simulink model "MAS_new"  (R2023a)
settings: Solver=VariableStepAuto  StartTime=0.0  StopTime=1  RelTol=1e-3
values from neighbouring files (symbols this model uses):
  abc_alpha_beta = sqrt(2/3) * [1, -1/2, -1/2 ... (first row only)    [main.m]
  Flux_1 = 1/(Msr^2 - Ls * Lr )  * [Rs*Lr, 0, -Rs*Msr, 0 ... (first row only)    [main.m]
  Flux_2 = 1/(Msr^2 - Ls * Lr )  * [0, 0, 0, 0 ... (first row only)    [main.m]
  frot = 0.01    [main.m]
  Inv_abc_alpha_beta = inv(abc_alpha_beta)    [main.m]
  Inv_Phi_Courant = inv(Phi_Courant)    [main.m]
  J = 0.025    [main.m]
  Lr = 0.194    [main.m]
  Ls = 0.182    [main.m]
  Msr = 0.182    [main.m]
  p = 2    [main.m]
  T_charge = 0    [main.m]
  Vn = 380    [main.m]
settings Model: Creator=philippecasteres  LastModifiedBy=philippecasteres

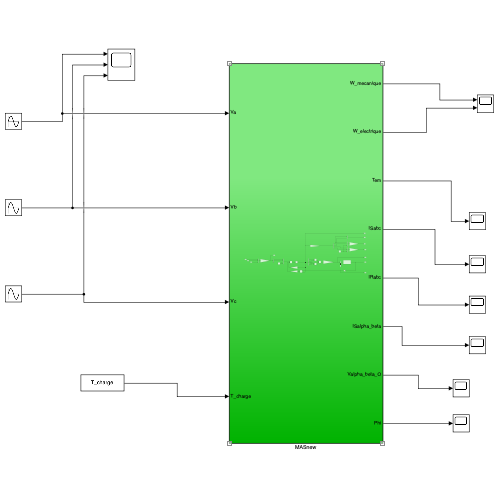
[thumbnail: Simulink's stored preview of the top-level diagram]
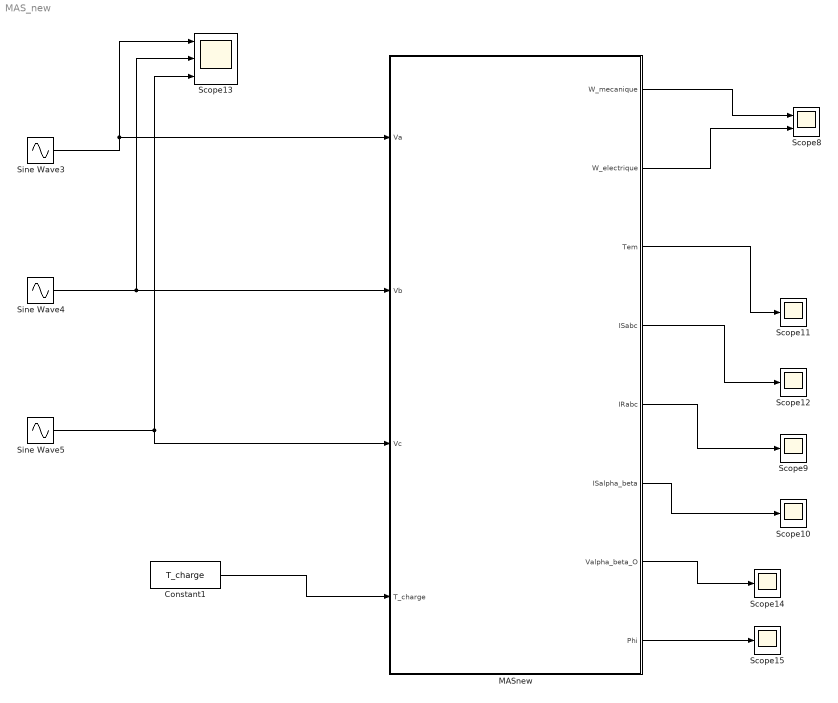
== system MAS_new ==
  Constant1 : Constant  Value=T_charge
  MASnew : Subsystem
  Scope{9..12,14..15} (6 alike) : Scope
  Scope13 : Scope  NumInputPorts=3
  Scope8 : Scope  NumInputPorts=2
  Sine Wave3 : Sin  Amplitude=Vn  Frequency=50*2*pi  SampleTime=0
  Sine Wave4 : Sin  Amplitude=Vn  Frequency=50*2*pi  Phase=-2*pi/3  SampleTime=0
  Sine Wave5 : Sin  Amplitude=Vn  Frequency=50*2*pi  Phase=-4*pi/3  SampleTime=0
  wires:
  MASnew/1(W_mecanique) -> Scope8/1
  MASnew/7(Valpha_beta_O) -> Scope14/1
  Sine Wave4/1 -> Scope13/2, MASnew/2(Vb)
  Sine Wave5/1 -> Scope13/3, MASnew/3(Vc)
  MASnew/6(ISalpha_beta) -> Scope10/1
  MASnew/8(Phi) -> Scope15/1
  MASnew/5(IRabc) -> Scope9/1
  MASnew/3(Tem) -> Scope11/1
  MASnew/4(ISabc) -> Scope12/1
  Sine Wave3/1 -> MASnew/1(Va), Scope13/1
  MASnew/2(W_electrique) -> Scope8/2
  Constant1/1 -> MASnew/4(T_charge)

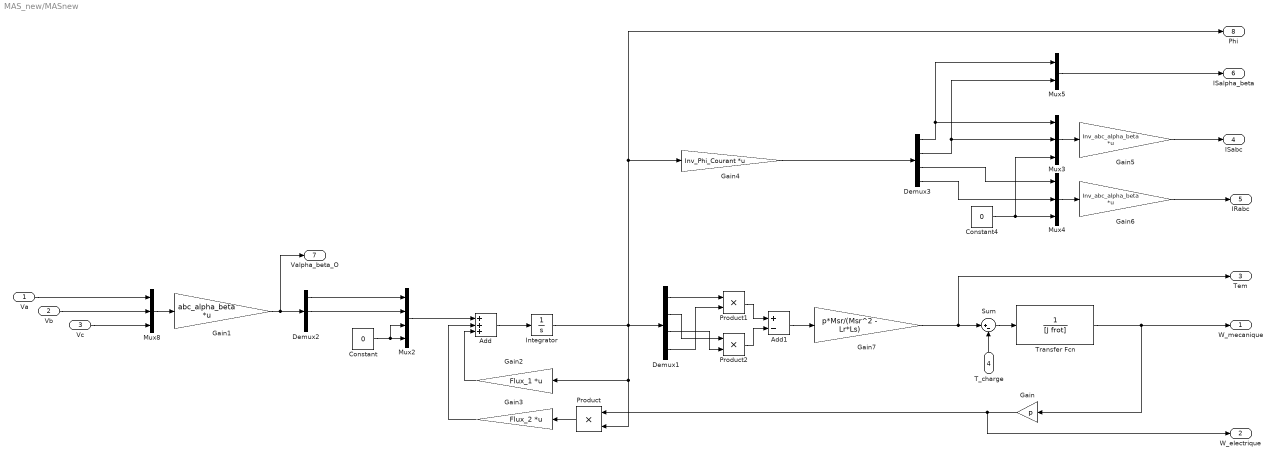
== system MAS_new/MASnew ==
  Va : Inport
  Vb : Inport  Port=2
  Vc : Inport  Port=3
  T_charge : Inport  Port=4
  Add : Sum  Inputs=+++
  Add1 : Sum  Inputs=+-
  Constant : Constant  Value=0
  Constant4 : Constant  Value=0
  Demux1 : Demux
  Demux2 : Demux  Outputs=3
  Demux3 : Demux
  Gain : Gain  Gain=p
  Gain1 : Gain  Gain=abc_alpha_beta  Multiplication=Matrix(K*u)
  Gain2 : Gain  Gain=Flux_1  Multiplication=Matrix(K*u)
  Gain3 : Gain  Gain=Flux_2  Multiplication=Matrix(K*u)
  Gain4 : Gain  Gain=Inv_Phi_Courant  Multiplication=Matrix(K*u)
  Gain5 : Gain  Gain=Inv_abc_alpha_beta  Multiplication=Matrix(K*u)
  Gain6 : Gain  Gain=Inv_abc_alpha_beta  Multiplication=Matrix(K*u)
  Gain7 : Gain  Gain=p*Msr/(Msr^2 - Lr*Ls)
  Integrator : Integrator
  Mux2 : Mux
  Mux3 : Mux  Inputs=3
  Mux4 : Mux  Inputs=3
  Mux5 : Mux  Inputs=2
  Mux8 : Mux  Inputs=3
  Product : Product
  Product1 : Product
  Product2 : Product
  Sum : Sum  Inputs=|+-
  Transfer Fcn : TransferFcn  Denominator=[J frot]
  W_mecanique : Outport
  W_electrique : Outport  Port=2
  Tem : Outport  Port=3
  ISabc : Outport  Port=4
  IRabc : Outport  Port=5
  ISalpha_beta : Outport  Port=6
  Valpha_beta_O : Outport  Port=7
  Phi : Outport  Port=8
  wires:
  Demux3/4 -> Mux4/2
  Demux3/2 -> Mux3/2, Mux5/2
  T_charge/1 -> Sum/2
  Demux3/1 -> Mux3/1, Mux5/1
  Va/1 -> Mux8/1
  Sum/1 -> Transfer Fcn/1
  Demux1/1 -> Product1/1
  Demux3/3 -> Mux4/1
  Gain7/1 -> Sum/1, Tem/1
  Transfer Fcn/1 -> Gain/1, W_mecanique/1
  Add/1 -> Integrator/1
  Vc/1 -> Mux8/3
  Vb/1 -> Mux8/2
  Product/1 -> Gain3/1
  Integrator/1 -> Gain2/1, Product/2, Demux1/1, Gain4/1, Phi/1
  Mux2/1 -> Add/1
  Mux3/1 -> Gain5/1
  Mux5/1 -> ISalpha_beta/1
  Gain1/1 -> Valpha_beta_O/1, Demux2/1
  Mux8/1 -> Gain1/1
  Demux2/1 -> Mux2/1
  Demux2/2 -> Mux2/2
  Constant/1 -> Mux2/4, Mux2/3
  Gain2/1 -> Add/3
  Gain4/1 -> Demux3/1
  Constant4/1 -> Mux4/3, Mux3/3
  Gain5/1 -> ISabc/1
  Mux4/1 -> Gain6/1
  Gain6/1 -> IRabc/1
  Product1/1 -> Add1/1
  Product2/1 -> Add1/2
  Add1/1 -> Gain7/1
  Gain/1 -> W_electrique/1, Product/1
  Gain3/1 -> Add/2
  Demux1/4 -> Product1/2
  Demux1/2 -> Product2/1
  Demux1/3 -> Product2/2
